simulink model "DAL_Sat_HW_ExtendedControl_photo"  (R2021b)
settings: Solver=FixedStepAuto  StartTime=0.0  StopTime=Inf  RelTol=1e-3  EnableMultiTasking=on
undefined symbols (not defined in the file): magnitude
libraries: arduinolib x12
settings Model: ExtModeTrigDuration=2  Creator=diego  LastModifiedBy=diego
settings OptimizationCC: EnhancedBackFolding=on  PassReuseOutputArgsAs=Individual arguments  ZeroExternalMemoryAtStartup=off  ZeroInternalMemoryAtStartup=off  MaxStackSize=64  OptimizeBlockOrder=speed  DifferentSizesBufferReuse=on  EfficientTunableParamExpr=on
settings DebuggingCC: ParameterTunabilityLossMsg=error
settings HardwareCC: ProdBitPerInt=16  ProdBitPerPointer=16  ProdBitPerSizeT=16  ProdBitPerPtrDiffT=16  ProdLargestAtomicFloat=None  ProdWordSize=8  ProdHWDeviceType=Atmel->AVR
settings SFSimCC: MATLABDynamicMemAlloc=off
settings RTWCC: Description=Embedded Coder  SystemTargetFile=ert.tlc  HardwareBoard=Arduino Uno  TemplateMakefile=ert_default_tmf  Toolchain=Arduino AVR  BuildConfiguration=Faster Runs
settings CodeAppCC: ForceParamTrailComments=on  IgnoreCustomStorageClasses=off  OperatorAnnotations=on  SimulinkDataObjDesc=on  SFDataObjDesc=on  InsertBlockDesc=on
settings ERTTargetCC: SupportContinuousTime=on  SupportVariableSizeSignals=on  ExtModeTransport=3  ExtModeStaticAlloc=on  ExtModeStaticAllocSize=250  ExtModeMexFile=ext_xcp  ExtModeIntrfLevel=Level2 - Open

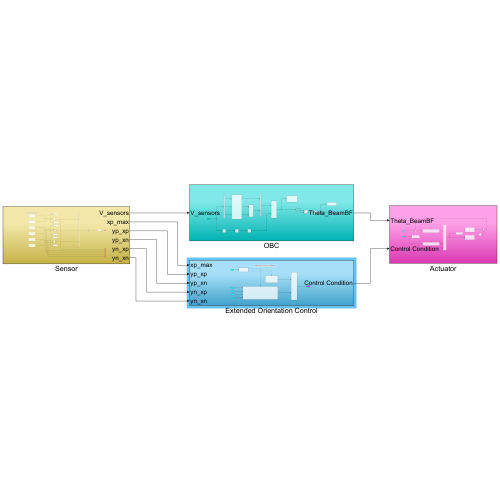
[thumbnail: Simulink's stored preview of the top-level diagram]
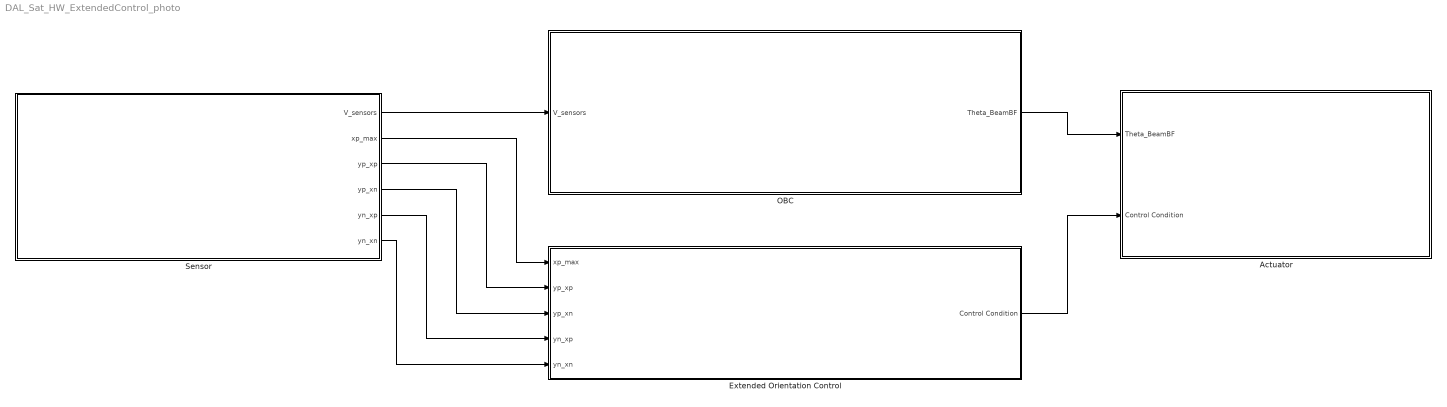
== system DAL_Sat_HW_ExtendedControl_photo ==
  Actuator : Subsystem
  Extended Orientation Control : Subsystem
  OBC : Subsystem
  Sensor : Subsystem
  wires:
  Sensor/1(V_sensors) -> OBC/1(V_sensors)
  OBC/1(Theta_BeamBF) -> Actuator/1(Theta_BeamBF)
  Sensor/2(xp_max) -> Extended Orientation Control/1(xp_max)
  Sensor/3(yp_xp) -> Extended Orientation Control/2(yp_xp)
  Sensor/4(yp_xn) -> Extended Orientation Control/3(yp_xn)
  Sensor/5(yn_xp) -> Extended Orientation Control/4(yn_xp)
  Sensor/6(yn_xn) -> Extended Orientation Control/5(yn_xn)
  Extended Orientation Control/1(Control Condition) -> Actuator/2(Control Condition)

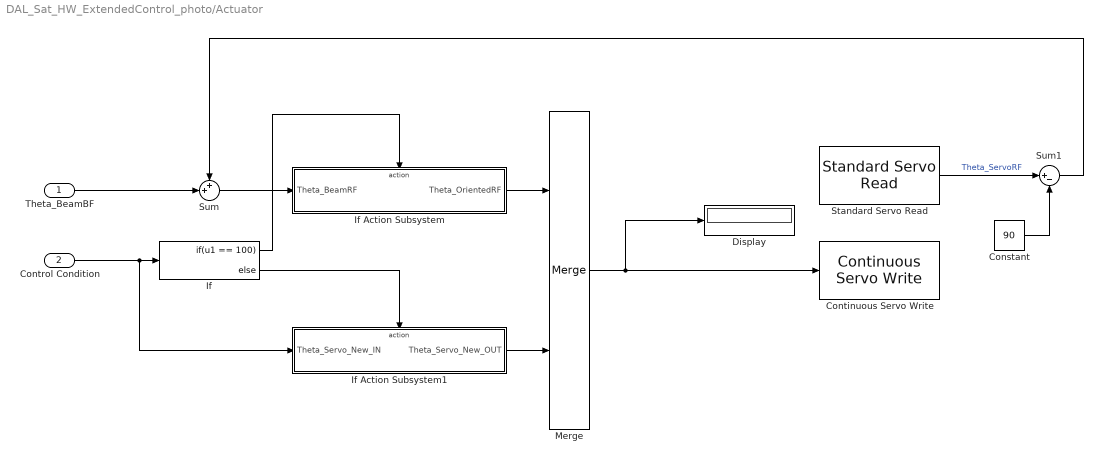
== system DAL_Sat_HW_ExtendedControl_photo/Actuator ==
  Theta_BeamBF : Inport
  Control Condition : Inport  Port=2
  Constant : Constant  Value=90
  Continuous Servo Write : arduinolib/Continuous Servo Write  pinNumber=9  ServoIndex=0  blockPlatform=ARDUINO
      settings: SourceProductBaseCode=ARDUINO
  Display : Display
  If : If  IfExpression=u1 == 100
  If Action Subsystem : Subsystem  TreatAsAtomicUnit=on
  If Action Subsystem1 : Subsystem  TreatAsAtomicUnit=on
  Merge : Merge
  Standard Servo Read : arduinolib/Standard Servo Read  pinNumber=9  SampleTime=0.1  ServoIndex=0  blockPlatform=ARDUINO
      settings: SourceProductBaseCode=ARDUINO
  Sum : Sum  Inputs=++|
  Sum1 : Sum  Inputs=|+-
  wires:
  Standard Servo Read/1 -> Sum1/1  "Theta_ServoRF"
  Theta_BeamBF/1 -> Sum/2
  Constant/1 -> Sum1/2
  Merge/1 -> Continuous Servo Write/1, Display/1
  Control Condition/1 -> If Action Subsystem1/1(Theta_Servo_New_IN), If/1
  If/1 -> If Action Subsystem/Action
  If/2 -> If Action Subsystem1/Action
  If Action Subsystem/1(Theta_OrientedRF) -> Merge/1
  If Action Subsystem1/1(Theta_Servo_New_OUT) -> Merge/2
  Sum/1 -> If Action Subsystem/1(Theta_BeamRF)
  Sum1/1 -> Sum/1

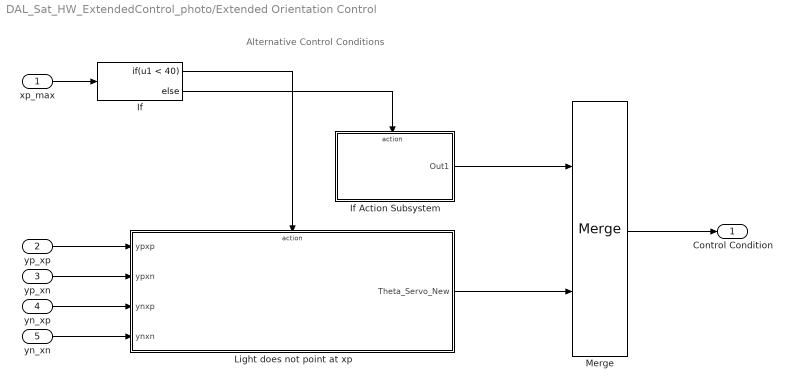
== system DAL_Sat_HW_ExtendedControl_photo/Extended Orientation Control ==
  note: Alternative Control Conditions
  xp_max : Inport
  yp_xp : Inport  Port=2
  yp_xn : Inport  Port=3
  yn_xp : Inport  Port=4
  yn_xn : Inport  Port=5
  If : If  IfExpression=u1 < 40
  If Action Subsystem : Subsystem  TreatAsAtomicUnit=on
  Light does not point at xp : Subsystem  TreatAsAtomicUnit=on
  Merge : Merge
  Control Condition : Outport
  wires:
  Merge/1 -> Control Condition/1
  yn_xp/1 -> Light does not point at xp/3(ynxp)
  yn_xn/1 -> Light does not point at xp/4(ynxn)
  xp_max/1 -> If/1
  If Action Subsystem/1(Out1) -> Merge/1
  If/2 -> If Action Subsystem/Action
  If/1 -> Light does not point at xp/Action
  Light does not point at xp/1(Theta_Servo_New) -> Merge/2
  yp_xp/1 -> Light does not point at xp/1(ypxp)
  yp_xn/1 -> Light does not point at xp/2(ypxn)

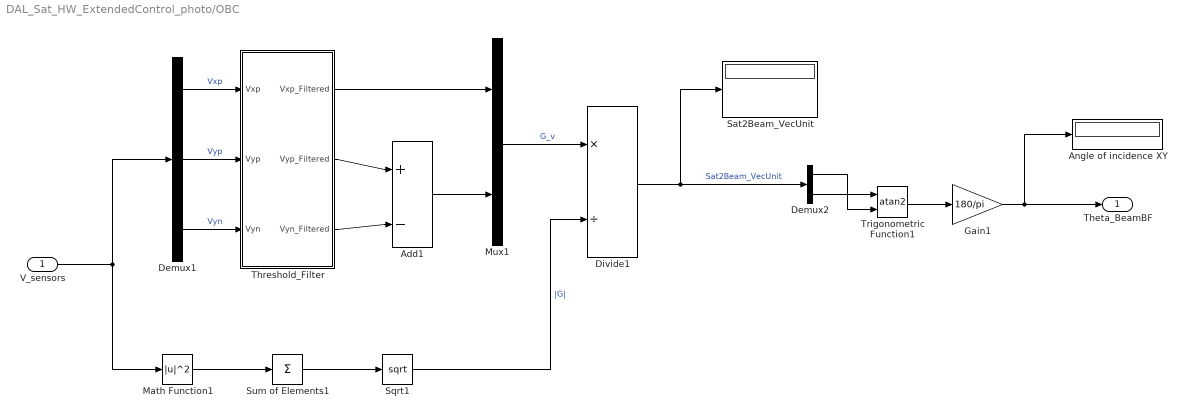
== system DAL_Sat_HW_ExtendedControl_photo/OBC ==
  V_sensors : Inport
  Add1 : Sum  Inputs=+|-
  Angle of incidence XY : Display
  Demux1 : Demux  Outputs=3
  Demux2 : Demux  Outputs=2
  Divide1 : Product  Inputs=*/
  Gain1 : Gain  Gain=180/pi
  Math Function1 : Math  Operator=magnitude^2  OutputSignalType=real  SaturateOnIntegerOverflow=on
  Mux1 : Mux  Inputs=2
  Sat2Beam_VecUnit : Display
  Sqrt1 : Sqrt  SaturateOnIntegerOverflow=on
  Sum of Elements1 : Sum  Inputs=+
  Threshold_Filter : Subsystem
  Trigonometric Function1 : Trigonometry  Operator=atan2
  Theta_BeamBF : Outport
  wires:
  Math Function1/1 -> Sum of Elements1/1
  Gain1/1 -> Theta_BeamBF/1, Angle of incidence XY/1
  Divide1/1 -> Demux2/1, Sat2Beam_VecUnit/1  "Sat2Beam_VecUnit"
  Demux2/2 -> Trigonometric Function1/1
  Add1/1 -> Mux1/2
  Sum of Elements1/1 -> Sqrt1/1
  Sqrt1/1 -> Divide1/2  "|G|"
  Mux1/1 -> Divide1/1  "G_v"
  Threshold_Filter/3(Vyn_Filtered) -> Add1/2
  Threshold_Filter/2(Vyp_Filtered) -> Add1/1
  Demux1/3 -> Threshold_Filter/3(Vyn)  "Vyn"
  V_sensors/1 -> Demux1/1, Math Function1/1
  Threshold_Filter/1(Vxp_Filtered) -> Mux1/1
  Demux2/1 -> Trigonometric Function1/2
  Demux1/1 -> Threshold_Filter/1(Vxp)  "Vxp"
  Trigonometric Function1/1 -> Gain1/1
  Demux1/2 -> Threshold_Filter/2(Vyp)  "Vyp"

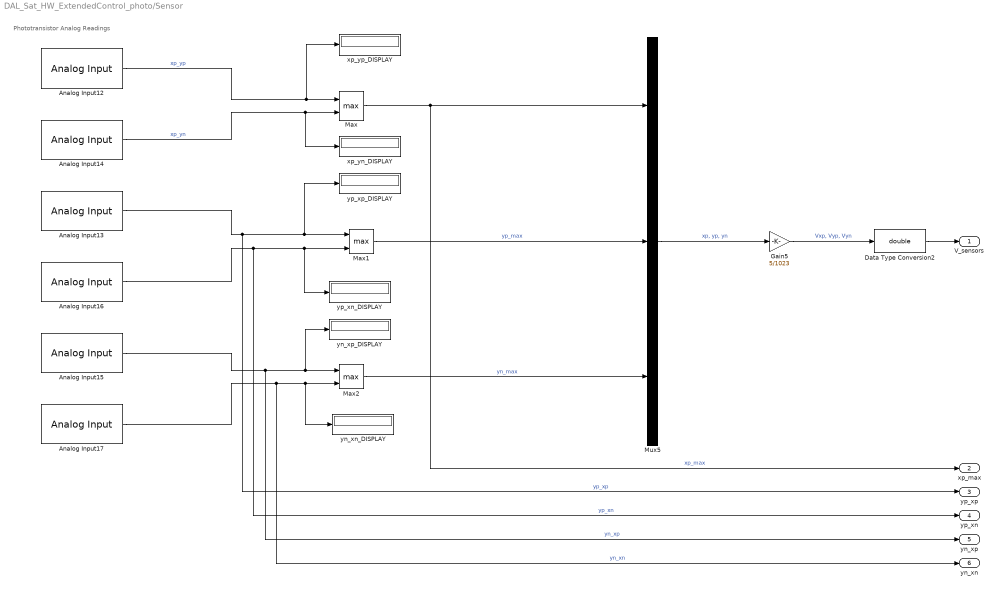
== system DAL_Sat_HW_ExtendedControl_photo/Sensor ==
  note: Phototransistor Analog Readings
  Analog Input12 : arduinolib/Analog Input  pinNumber=2  ReadResultsOnly=off  ConversionTriggerSource=Software  ExternalTriggerType=uint32( 0 )  OutputDataType=uint16  EnableConversionCompleteNotify=off  EnableOuputStatus=off  SampleTime=-1  blockPlatform=arduino
  Analog Input13 : arduinolib/Analog Input  pinNumber=1  ReadResultsOnly=off  ConversionTriggerSource=Software  ExternalTriggerType=uint32( 0 )  OutputDataType=uint16  EnableConversionCompleteNotify=off  EnableOuputStatus=off  SampleTime=-1  blockPlatform=arduino
  Analog Input14 : arduinolib/Analog Input  pinNumber=3  ReadResultsOnly=off  ConversionTriggerSource=Software  ExternalTriggerType=uint32( 0 )  OutputDataType=uint16  EnableConversionCompleteNotify=off  EnableOuputStatus=off  SampleTime=-1  blockPlatform=arduino
  Analog Input15 : arduinolib/Analog Input  pinNumber=4  ReadResultsOnly=off  ConversionTriggerSource=Software  ExternalTriggerType=uint32( 0 )  OutputDataType=uint16  EnableConversionCompleteNotify=off  EnableOuputStatus=off  SampleTime=-1  blockPlatform=arduino
  Analog Input16 : arduinolib/Analog Input  pinNumber=0  ReadResultsOnly=off  ConversionTriggerSource=Software  ExternalTriggerType=uint32( 0 )  OutputDataType=uint16  EnableConversionCompleteNotify=off  EnableOuputStatus=off  SampleTime=-1  blockPlatform=arduino
  Analog Input17 : arduinolib/Analog Input  pinNumber=5  ReadResultsOnly=off  ConversionTriggerSource=Software  ExternalTriggerType=uint32( 0 )  OutputDataType=uint16  EnableConversionCompleteNotify=off  EnableOuputStatus=off  SampleTime=-1  blockPlatform=arduino
  Data Type Conversion2 : DataTypeConversion  OutDataTypeStr=double
  Gain5 : Gain  Gain=5/1023
  Max : MinMax  Function=max  Inputs=2
  Max1 : MinMax  Function=max  Inputs=2
  Max2 : MinMax  Function=max  Inputs=2
  Mux5 : Mux  Inputs=3
  xp_yn_DISPLAY : Display
  xp_yp_DISPLAY : Display
  yn_xn_DISPLAY : Display
  yn_xp_DISPLAY : Display
  yp_xn_DISPLAY : Display
  yp_xp_DISPLAY : Display
  V_sensors : Outport
  xp_max : Outport  Port=2
  yp_xp : Outport  Port=3
  yp_xn : Outport  Port=4
  yn_xp : Outport  Port=5
  yn_xn : Outport  Port=6
  wires:
  Analog Input12/1 -> Max/1, xp_yp_DISPLAY/1  "xp_yp"
  Analog Input14/1 -> Max/2, xp_yn_DISPLAY/1  "xp_yn"
  Analog Input13/1 -> yp_xp/1, Max1/1, yp_xp_DISPLAY/1  "yp_xp"
  Max2/1 -> Mux5/3  "yn_max"
  Max/1 -> xp_max/1, Mux5/1  "xp_max"
  Analog Input15/1 -> yn_xp/1, Max2/1, yn_xp_DISPLAY/1  "yn_xp"
  Analog Input16/1 -> yp_xn/1, Max1/2, yp_xn_DISPLAY/1  "yp_xn"
  Analog Input17/1 -> yn_xn/1, Max2/2, yn_xn_DISPLAY/1  "yn_xn"
  Max1/1 -> Mux5/2  "yp_max"
  Mux5/1 -> Gain5/1  "xp, yp, yn"
  Gain5/1 -> Data Type Conversion2/1  "Vxp, Vyp, Vyn"
  Data Type Conversion2/1 -> V_sensors/1

== system DAL_Sat_HW_ExtendedControl_photo/Actuator/If Action Subsystem ==
  Theta_BeamRF : Inport
  Action Port : ActionPort  ActionPortLabel=if(u1 == 100)
  Abs1 : Abs
  If : If  IfExpression=u1 > 90
  If Action Subsystem1 : Subsystem  TreatAsAtomicUnit=on
  If Action Subsystem4 : Subsystem  TreatAsAtomicUnit=on
  Merge1 : Merge
  Theta_OrientedRF : Outport
  wires:
  If Action Subsystem4/1(Theta_OrientedRF) -> Merge1/2
  If/1 -> If Action Subsystem1/Action
  Abs1/1 -> If/1
  If/2 -> If Action Subsystem4/Action
  Theta_BeamRF/1 -> If Action Subsystem1/1(Theta_Beam	RF), Abs1/1, If Action Subsystem4/1(Theta_BeamRF)
  Merge1/1 -> Theta_OrientedRF/1
  If Action Subsystem1/1(Theta_OrientedRF) -> Merge1/1

== system DAL_Sat_HW_ExtendedControl_photo/Actuator/If Action Subsystem1 ==
  Theta_Servo_New_IN : Inport
  Action Port : ActionPort  ActionPortLabel=else
  Theta_Servo_New_OUT : Outport
  wires:
  Theta_Servo_New_IN/1 -> Theta_Servo_New_OUT/1

== system DAL_Sat_HW_ExtendedControl_photo/Extended Orientation Control/If Action Subsystem ==
  Action Port : ActionPort  ActionPortLabel=else
  Nominal Control Condition : Constant  Value=100
  Out1 : Outport
  wires:
  Nominal Control Condition/1 -> Out1/1

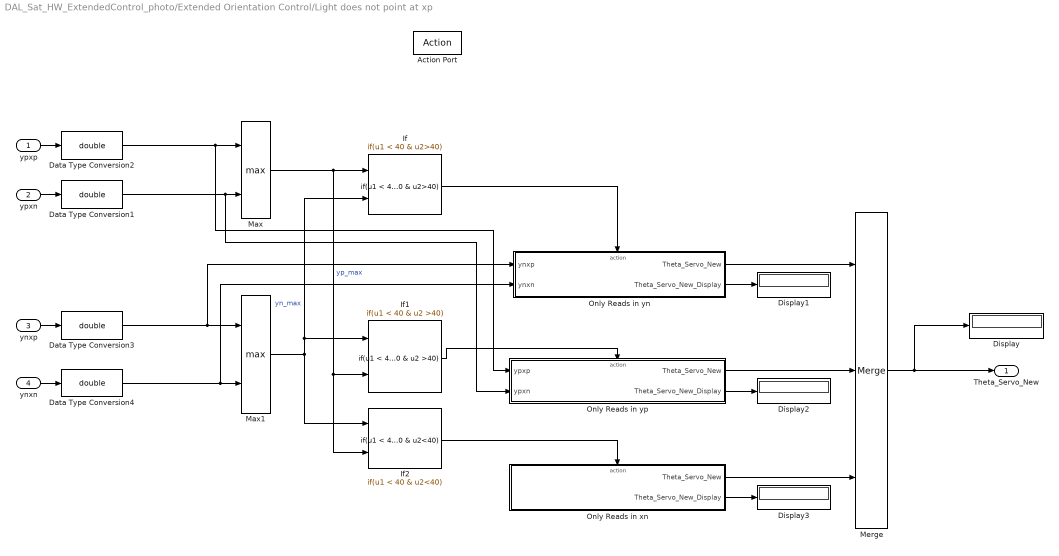
== system DAL_Sat_HW_ExtendedControl_photo/Extended Orientation Control/Light does not point at xp ==
  ypxp : Inport
  ypxn : Inport  Port=2
  ynxp : Inport  Port=3
  ynxn : Inport  Port=4
  Action Port : ActionPort  ActionPortLabel=if(u1 < 40)
  Data Type Conversion{1..4} (4 alike) : DataTypeConversion  OutDataTypeStr=double
  Display{,1..3} (4 alike) : Display
  If : If  NumInputs=2  IfExpression=u1 < 40 & u2>40  ShowElse=off
  If1 : If  NumInputs=2  IfExpression=u1 < 40 & u2 >40  ShowElse=off
  If2 : If  NumInputs=2  IfExpression=u1 < 40 & u2<40  ShowElse=off
  Max : MinMax  Function=max  Inputs=2
  Max1 : MinMax  Function=max  Inputs=2
  Merge : Merge  Inputs=3
  Only Reads in xn : Subsystem  TreatAsAtomicUnit=on
  Only Reads in yn : Subsystem  TreatAsAtomicUnit=on
  Only Reads in yp : Subsystem  TreatAsAtomicUnit=on
  Theta_Servo_New : Outport
  wires:
  Max/1 -> If/1, If2/2, If1/2  "yp_max"
  Max1/1 -> If2/1, If1/1, If/2  "yn_max"
  Only Reads in yn/1(Theta_Servo_New) -> Merge/1
  Only Reads in yp/1(Theta_Servo_New) -> Merge/2
  Merge/1 -> Display/1, Theta_Servo_New/1
  If/1 -> Only Reads in yn/Action
  If1/1 -> Only Reads in yp/Action
  If2/1 -> Only Reads in xn/Action
  Only Reads in xn/1(Theta_Servo_New) -> Merge/3
  Only Reads in yn/2(Theta_Servo_New_Display) -> Display1/1
  Only Reads in yp/2(Theta_Servo_New_Display) -> Display2/1
  Only Reads in xn/2(Theta_Servo_New_Display) -> Display3/1
  Data Type Conversion2/1 -> Max/1, Only Reads in yp/1(ypxp)
  Data Type Conversion1/1 -> Max/2, Only Reads in yp/2(ypxn)
  Data Type Conversion3/1 -> Max1/1, Only Reads in yn/1(ynxp)
  ypxn/1 -> Data Type Conversion1/1
  ypxp/1 -> Data Type Conversion2/1
  ynxn/1 -> Data Type Conversion4/1
  ynxp/1 -> Data Type Conversion3/1
  Data Type Conversion4/1 -> Only Reads in yn/2(ynxn), Max1/2

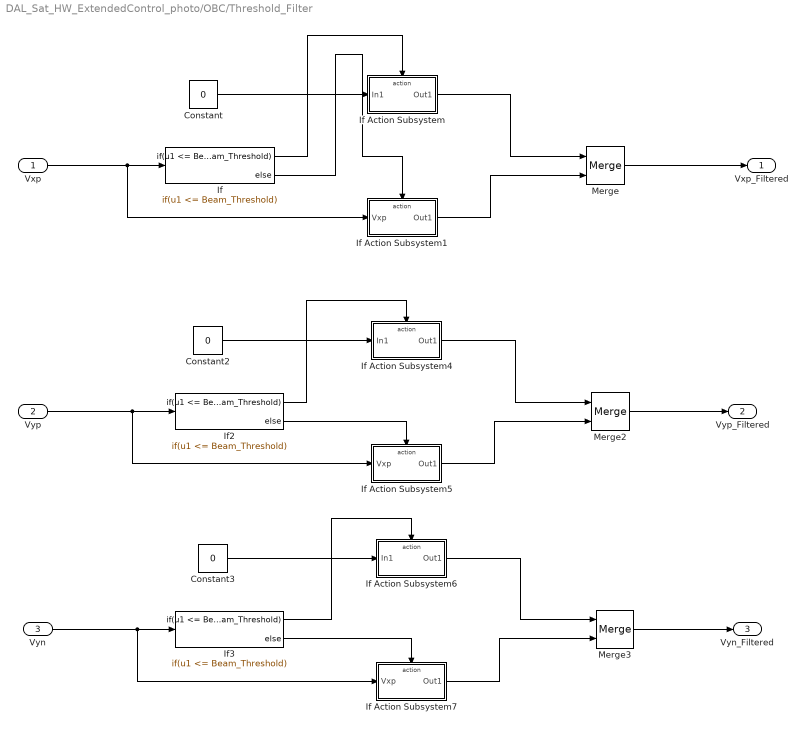
== system DAL_Sat_HW_ExtendedControl_photo/OBC/Threshold_Filter ==
  Vxp : Inport
  Vyp : Inport  Port=2
  Vyn : Inport  Port=3
  Constant : Constant  Value=0
  Constant2 : Constant  Value=0
  Constant3 : Constant  Value=0
  If : If  IfExpression=u1 <= Beam_Threshold
  If Action Subsystem : Subsystem  TreatAsAtomicUnit=on
  If Action Subsystem1 : Subsystem  TreatAsAtomicUnit=on
  If Action Subsystem4 : Subsystem  TreatAsAtomicUnit=on
  If Action Subsystem5 : Subsystem  TreatAsAtomicUnit=on
  If Action Subsystem6 : Subsystem  TreatAsAtomicUnit=on
  If Action Subsystem7 : Subsystem  TreatAsAtomicUnit=on
  If2 : If  IfExpression=u1 <= Beam_Threshold
  If3 : If  IfExpression=u1 <= Beam_Threshold
  Merge : Merge
  Merge2 : Merge
  Merge3 : Merge
  Vxp_Filtered : Outport
  Vyp_Filtered : Outport  Port=2
  Vyn_Filtered : Outport  Port=3
  wires:
  Vxp/1 -> If Action Subsystem1/1(Vxp), If/1
  If/1 -> If Action Subsystem/Action
  If Action Subsystem/1(Out1) -> Merge/1
  If/2 -> If Action Subsystem1/Action
  If Action Subsystem1/1(Out1) -> Merge/2
  Merge/1 -> Vxp_Filtered/1
  Constant/1 -> If Action Subsystem/1(In1)
  Vyp/1 -> If2/1, If Action Subsystem5/1(Vxp)
  If2/2 -> If Action Subsystem5/Action
  If2/1 -> If Action Subsystem4/Action
  If Action Subsystem4/1(Out1) -> Merge2/1
  If Action Subsystem5/1(Out1) -> Merge2/2
  Constant2/1 -> If Action Subsystem4/1(In1)
  Merge2/1 -> Vyp_Filtered/1
  Vyn/1 -> If3/1, If Action Subsystem7/1(Vxp)
  Merge3/1 -> Vyn_Filtered/1
  If Action Subsystem7/1(Out1) -> Merge3/2
  If3/2 -> If Action Subsystem7/Action
  If Action Subsystem6/1(Out1) -> Merge3/1
  Constant3/1 -> If Action Subsystem6/1(In1)
  If3/1 -> If Action Subsystem6/Action

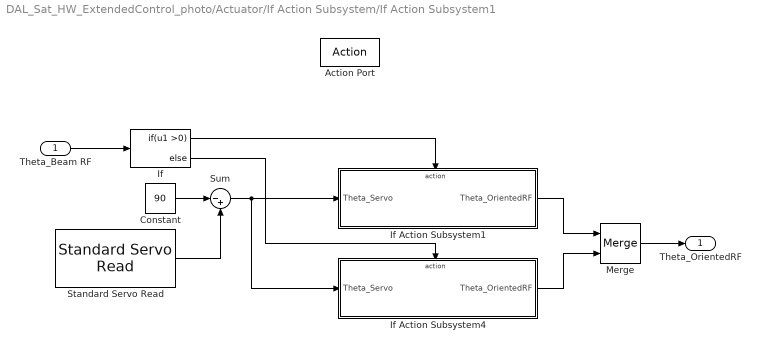
== system DAL_Sat_HW_ExtendedControl_photo/Actuator/If Action Subsystem/If Action Subsystem1 ==
  Theta_Beam	RF : Inport
  Action Port : ActionPort  ActionPortLabel=if(u1 > 90)
  Constant : Constant  Value=90
  If : If  IfExpression=u1 >0
  If Action Subsystem1 : Subsystem  TreatAsAtomicUnit=on
  If Action Subsystem4 : Subsystem  TreatAsAtomicUnit=on
  Merge : Merge
  Standard Servo Read : arduinolib/Standard Servo Read  pinNumber=9  SampleTime=0.1  ServoIndex=0  blockPlatform=ARDUINO
      settings: SourceProductBaseCode=ARDUINO
  Sum : Sum  Inputs=|-+
  Theta_OrientedRF : Outport
  wires:
  If/1 -> If Action Subsystem1/Action
  If/2 -> If Action Subsystem4/Action
  If Action Subsystem1/1(Theta_OrientedRF) -> Merge/1
  If Action Subsystem4/1(Theta_OrientedRF) -> Merge/2
  Merge/1 -> Theta_OrientedRF/1
  Theta_Beam	RF/1 -> If/1
  Standard Servo Read/1 -> Sum/2
  Sum/1 -> If Action Subsystem4/1(Theta_Servo), If Action Subsystem1/1(Theta_Servo)
  Constant/1 -> Sum/1

== system DAL_Sat_HW_ExtendedControl_photo/Actuator/If Action Subsystem/If Action Subsystem4 ==
  Theta_BeamRF : Inport
  Action Port : ActionPort  ActionPortLabel=else
  Theta_OrientedRF : Outport
  wires:
  Theta_BeamRF/1 -> Theta_OrientedRF/1

== system DAL_Sat_HW_ExtendedControl_photo/Extended Orientation Control/Light does not point at xp/Only Reads in xn ==
  Action Port : ActionPort  ActionPortLabel=if(u1 < 40 & u2<40)
  Constant : Constant  Value=90
  Data Type Conversion : DataTypeConversion  OutDataTypeStr=double
  Standard Servo Read : arduinolib/Standard Servo Read  pinNumber=9  SampleTime=0.1  ServoIndex=0  blockPlatform=ARDUINO
      settings: SourceProductBaseCode=ARDUINO
  Sum : Sum  Inputs=|+-
  Theta_Servo_New : Outport
  Theta_Servo_New_Display : Outport  Port=2
  wires:
  Data Type Conversion/1 -> Theta_Servo_New_Display/1, Theta_Servo_New/1
  Standard Servo Read/1 -> Sum/1
  Sum/1 -> Data Type Conversion/1
  Constant/1 -> Sum/2

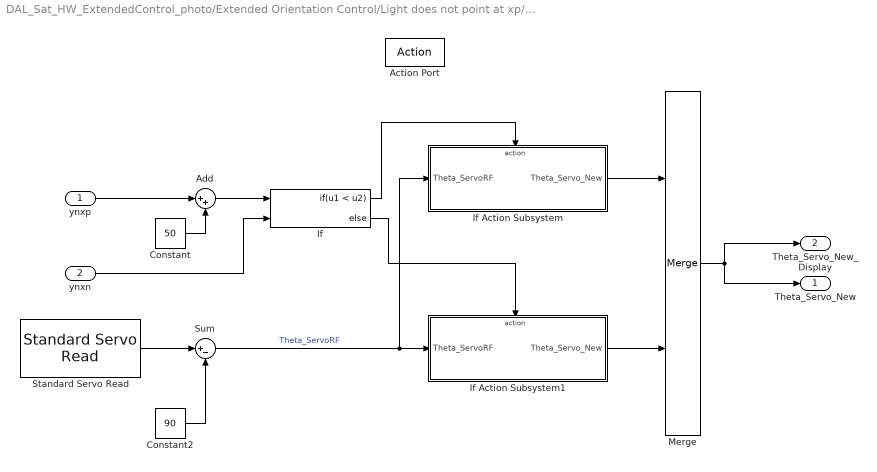
== system DAL_Sat_HW_ExtendedControl_photo/Extended Orientation Control/Light does not point at xp/Only Reads in yn ==
  ynxp : Inport
  ynxn : Inport  Port=2
  Action Port : ActionPort  ActionPortLabel=if(u1 < 40 & u2>40)
  Add : Sum  Inputs=|++
  Constant : Constant  Value=50
  Constant2 : Constant  Value=90
  If : If  NumInputs=2  IfExpression=u1 < u2
  If Action Subsystem : Subsystem  TreatAsAtomicUnit=on
  If Action Subsystem1 : Subsystem  TreatAsAtomicUnit=on
  Merge : Merge
  Standard Servo Read : arduinolib/Standard Servo Read  pinNumber=9  SampleTime=0.1  ServoIndex=0  blockPlatform=ARDUINO
      settings: SourceProductBaseCode=ARDUINO
  Sum : Sum  Inputs=|+-
  Theta_Servo_New : Outport
  Theta_Servo_New_Display : Outport  Port=2
  wires:
  ynxp/1 -> Add/1
  Constant/1 -> Add/2
  Add/1 -> If/1
  ynxn/1 -> If/2
  If/1 -> If Action Subsystem/Action
  If/2 -> If Action Subsystem1/Action
  Merge/1 -> Theta_Servo_New/1, Theta_Servo_New_Display/1
  Standard Servo Read/1 -> Sum/1
  Sum/1 -> If Action Subsystem1/1(Theta_ServoRF), If Action Subsystem/1(Theta_ServoRF)  "Theta_ServoRF"
  Constant2/1 -> Sum/2
  If Action Subsystem/1(Theta_Servo_New) -> Merge/1
  If Action Subsystem1/1(Theta_Servo_New) -> Merge/2

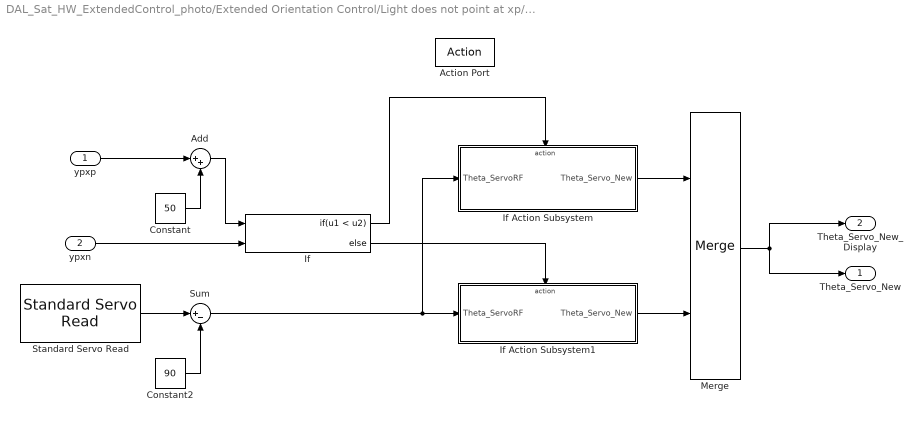
== system DAL_Sat_HW_ExtendedControl_photo/Extended Orientation Control/Light does not point at xp/Only Reads in yp ==
  ypxp : Inport
  ypxn : Inport  Port=2
  Action Port : ActionPort  ActionPortLabel=if(u1 < 40 & u2 >40)
  Add : Sum  Inputs=|++
  Constant : Constant  Value=50
  Constant2 : Constant  Value=90
  If : If  NumInputs=2  IfExpression=u1 < u2
  If Action Subsystem : Subsystem  TreatAsAtomicUnit=on
  If Action Subsystem1 : Subsystem  TreatAsAtomicUnit=on
  Merge : Merge
  Standard Servo Read : arduinolib/Standard Servo Read  pinNumber=9  SampleTime=0.1  ServoIndex=0  blockPlatform=ARDUINO
      settings: SourceProductBaseCode=ARDUINO
  Sum : Sum  Inputs=|+-
  Theta_Servo_New : Outport
  Theta_Servo_New_Display : Outport  Port=2
  wires:
  ypxp/1 -> Add/1
  Constant/1 -> Add/2
  Add/1 -> If/1
  ypxn/1 -> If/2
  If/1 -> If Action Subsystem/Action
  If/2 -> If Action Subsystem1/Action
  Merge/1 -> Theta_Servo_New/1, Theta_Servo_New_Display/1
  Sum/1 -> If Action Subsystem/1(Theta_ServoRF), If Action Subsystem1/1(Theta_ServoRF)
  Standard Servo Read/1 -> Sum/1
  Constant2/1 -> Sum/2
  If Action Subsystem/1(Theta_Servo_New) -> Merge/1
  If Action Subsystem1/1(Theta_Servo_New) -> Merge/2

== system DAL_Sat_HW_ExtendedControl_photo/OBC/Threshold_Filter/If Action Subsystem ==
  In1 : Inport
  Action Port : ActionPort  ActionPortLabel=if(u1 <= Beam_Threshold)
  Out1 : Outport
  wires:
  In1/1 -> Out1/1

== system DAL_Sat_HW_ExtendedControl_photo/OBC/Threshold_Filter/If Action Subsystem1 ==
  Vxp : Inport
  Action Port : ActionPort  ActionPortLabel=else
  Out1 : Outport
  wires:
  Vxp/1 -> Out1/1

== system DAL_Sat_HW_ExtendedControl_photo/OBC/Threshold_Filter/If Action Subsystem4 ==
  In1 : Inport
  Action Port : ActionPort  ActionPortLabel=if(u1 <= Beam_Threshold)
  Out1 : Outport
  wires:
  In1/1 -> Out1/1

== system DAL_Sat_HW_ExtendedControl_photo/OBC/Threshold_Filter/If Action Subsystem5 ==
  Vxp : Inport
  Action Port : ActionPort  ActionPortLabel=else
  Out1 : Outport
  wires:
  Vxp/1 -> Out1/1

== system DAL_Sat_HW_ExtendedControl_photo/OBC/Threshold_Filter/If Action Subsystem6 ==
  In1 : Inport
  Action Port : ActionPort  ActionPortLabel=if(u1 <= Beam_Threshold)
  Out1 : Outport
  wires:
  In1/1 -> Out1/1

== system DAL_Sat_HW_ExtendedControl_photo/OBC/Threshold_Filter/If Action Subsystem7 ==
  Vxp : Inport
  Action Port : ActionPort  ActionPortLabel=else
  Out1 : Outport
  wires:
  Vxp/1 -> Out1/1

== system DAL_Sat_HW_ExtendedControl_photo/Actuator/If Action Subsystem/If Action Subsystem1/If Action Subsystem1 ==
  Theta_Servo : Inport
  Action Port : ActionPort  ActionPortLabel=if(u1 >0)
  Constant : Constant  Value=5
  Subtract : Sum  Inputs=+-
  Theta_OrientedRF : Outport
  wires:
  Subtract/1 -> Theta_OrientedRF/1
  Theta_Servo/1 -> Subtract/1
  Constant/1 -> Subtract/2

== system DAL_Sat_HW_ExtendedControl_photo/Actuator/If Action Subsystem/If Action Subsystem1/If Action Subsystem4 ==
  Theta_Servo : Inport
  Action Port : ActionPort  ActionPortLabel=else
  Constant : Constant  Value=5
  Subtract : Sum
  Theta_OrientedRF : Outport
  wires:
  Theta_Servo/1 -> Subtract/1
  Constant/1 -> Subtract/2
  Subtract/1 -> Theta_OrientedRF/1

== system DAL_Sat_HW_ExtendedControl_photo/Extended Orientation Control/Light does not point at xp/Only Reads in yn/If Action Subsystem ==
  Theta_ServoRF : Inport
  Action Port : ActionPort  ActionPortLabel=if(u1 < u2)
  If : If  IfExpression=u1 >= 86
  If Action Subsystem : Subsystem  TreatAsAtomicUnit=on
  If Action Subsystem1 : Subsystem  TreatAsAtomicUnit=on
  Merge : Merge
  Theta_Servo_New : Outport
  wires:
  Theta_ServoRF/1 -> If Action Subsystem1/1(Theta_Servo_Old), If/1
  If/2 -> If Action Subsystem1/Action
  If Action Subsystem/1(Theta_Servo_New) -> Merge/1
  If Action Subsystem1/1(Theta_Servo_New) -> Merge/2
  Merge/1 -> Theta_Servo_New/1
  If/1 -> If Action Subsystem/Action

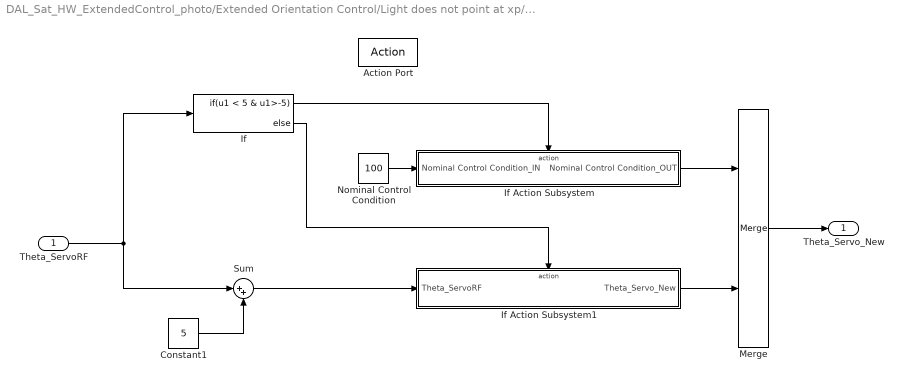
== system DAL_Sat_HW_ExtendedControl_photo/Extended Orientation Control/Light does not point at xp/Only Reads in yn/If Action Subsystem1 ==
  Theta_ServoRF : Inport
  Action Port : ActionPort  ActionPortLabel=else
  Constant1 : Constant  Value=5
  If : If  IfExpression=u1 < 5 & u1>-5
  If Action Subsystem : Subsystem  TreatAsAtomicUnit=on
  If Action Subsystem1 : Subsystem  TreatAsAtomicUnit=on
  Merge : Merge
  Nominal Control Condition : Constant  Value=100
  Sum : Sum  Inputs=|++
  Theta_Servo_New : Outport
  wires:
  If/1 -> If Action Subsystem/Action
  Nominal Control Condition/1 -> If Action Subsystem/1(Nominal Control Condition_IN)
  If/2 -> If Action Subsystem1/Action
  If Action Subsystem/1(Nominal Control Condition_OUT) -> Merge/1
  If Action Subsystem1/1(Theta_Servo_New) -> Merge/2
  Merge/1 -> Theta_Servo_New/1
  Sum/1 -> If Action Subsystem1/1(Theta_ServoRF)
  Theta_ServoRF/1 -> Sum/1, If/1
  Constant1/1 -> Sum/2

== system DAL_Sat_HW_ExtendedControl_photo/Extended Orientation Control/Light does not point at xp/Only Reads in yp/If Action Subsystem ==
  Theta_ServoRF : Inport
  Action Port : ActionPort  ActionPortLabel=if(u1 < u2)
  If : If  IfExpression=u1 <= -86
  If Action Subsystem : Subsystem  TreatAsAtomicUnit=on
  If Action Subsystem1 : Subsystem  TreatAsAtomicUnit=on
  Merge : Merge
  Theta_Servo_New : Outport
  wires:
  Theta_ServoRF/1 -> If Action Subsystem1/1(Theta_ServoRF), If/1
  If Action Subsystem/1(Theta_Servo_New) -> Merge/1
  If Action Subsystem1/1(Theta_Servo_New) -> Merge/2
  Merge/1 -> Theta_Servo_New/1
  If/2 -> If Action Subsystem1/Action
  If/1 -> If Action Subsystem/Action

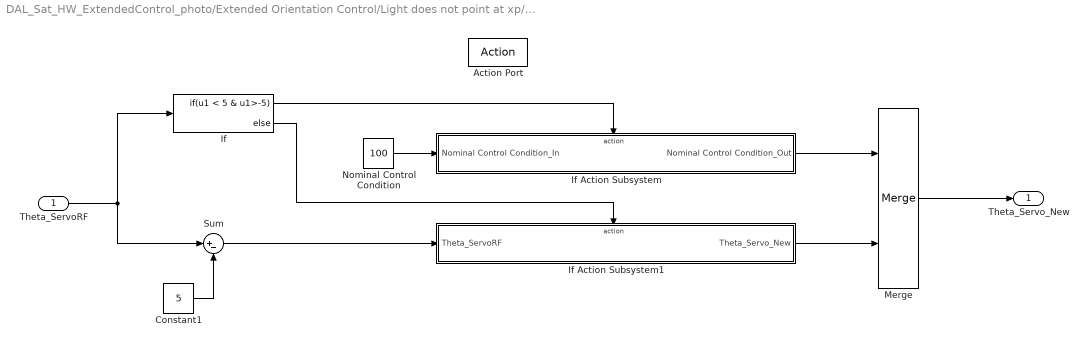
== system DAL_Sat_HW_ExtendedControl_photo/Extended Orientation Control/Light does not point at xp/Only Reads in yp/If Action Subsystem1 ==
  Theta_ServoRF : Inport
  Action Port : ActionPort  ActionPortLabel=else
  Constant1 : Constant  Value=5
  If : If  IfExpression=u1 < 5 & u1>-5
  If Action Subsystem : Subsystem  TreatAsAtomicUnit=on
  If Action Subsystem1 : Subsystem  TreatAsAtomicUnit=on
  Merge : Merge
  Nominal Control Condition : Constant  Value=100
  Sum : Sum  Inputs=|+-
  Theta_Servo_New : Outport
  wires:
  Merge/1 -> Theta_Servo_New/1
  Theta_ServoRF/1 -> Sum/1, If/1
  If/1 -> If Action Subsystem/Action
  If/2 -> If Action Subsystem1/Action
  If Action Subsystem1/1(Theta_Servo_New) -> Merge/2
  Nominal Control Condition/1 -> If Action Subsystem/1(Nominal Control Condition_In)
  If Action Subsystem/1(Nominal Control Condition_Out) -> Merge/1
  Sum/1 -> If Action Subsystem1/1(Theta_ServoRF)
  Constant1/1 -> Sum/2

== system DAL_Sat_HW_ExtendedControl_photo/Extended Orientation Control/Light does not point at xp/Only Reads in yn/If Action Subsystem/If Action Subsystem ==
  Action Port : ActionPort  ActionPortLabel=if(u1 >= 86)
  Constant : Constant  Value=-90
  Theta_Servo_New : Outport
  wires:
  Constant/1 -> Theta_Servo_New/1

== system DAL_Sat_HW_ExtendedControl_photo/Extended Orientation Control/Light does not point at xp/Only Reads in yn/If Action Subsystem/If Action Subsystem1 ==
  Theta_Servo_Old : Inport
  Action Port : ActionPort  ActionPortLabel=else
  Add : Sum
  Constant : Constant  Value=5
  Theta_Servo_New : Outport
  wires:
  Theta_Servo_Old/1 -> Add/1
  Add/1 -> Theta_Servo_New/1
  Constant/1 -> Add/2

== system DAL_Sat_HW_ExtendedControl_photo/Extended Orientation Control/Light does not point at xp/Only Reads in yn/If Action Subsystem1/If Action Subsystem ==
  Nominal Control Condition_IN : Inport
  Action Port : ActionPort  ActionPortLabel=if(u1 < 5 & u1>-5)
  Nominal Control Condition_OUT : Outport
  wires:
  Nominal Control Condition_IN/1 -> Nominal Control Condition_OUT/1

== system DAL_Sat_HW_ExtendedControl_photo/Extended Orientation Control/Light does not point at xp/Only Reads in yn/If Action Subsystem1/If Action Subsystem1 ==
  Theta_ServoRF : Inport
  Action Port : ActionPort  ActionPortLabel=else
  Theta_Servo_New : Outport
  wires:
  Theta_ServoRF/1 -> Theta_Servo_New/1

== system DAL_Sat_HW_ExtendedControl_photo/Extended Orientation Control/Light does not point at xp/Only Reads in yp/If Action Subsystem/If Action Subsystem ==
  Action Port : ActionPort  ActionPortLabel=if(u1 <= -86)
  Constant : Constant  Value=90
  Theta_Servo_New : Outport
  wires:
  Constant/1 -> Theta_Servo_New/1

== system DAL_Sat_HW_ExtendedControl_photo/Extended Orientation Control/Light does not point at xp/Only Reads in yp/If Action Subsystem/If Action Subsystem1 ==
  Theta_ServoRF : Inport
  Action Port : ActionPort  ActionPortLabel=else
  Add : Sum  Inputs=+-
  Constant : Constant  Value=5
  Theta_Servo_New : Outport
  wires:
  Theta_ServoRF/1 -> Add/1
  Add/1 -> Theta_Servo_New/1
  Constant/1 -> Add/2

== system DAL_Sat_HW_ExtendedControl_photo/Extended Orientation Control/Light does not point at xp/Only Reads in yp/If Action Subsystem1/If Action Subsystem ==
  Nominal Control Condition_In : Inport
  Action Port : ActionPort  ActionPortLabel=if(u1 < 5 & u1>-5)
  Nominal Control Condition_Out : Outport
  wires:
  Nominal Control Condition_In/1 -> Nominal Control Condition_Out/1

== system DAL_Sat_HW_ExtendedControl_photo/Extended Orientation Control/Light does not point at xp/Only Reads in yp/If Action Subsystem1/If Action Subsystem1 ==
  Theta_ServoRF : Inport
  Action Port : ActionPort  ActionPortLabel=else
  Theta_Servo_New : Outport
  wires:
  Theta_ServoRF/1 -> Theta_Servo_New/1
